simulink subsystem "currentControl"  (R2023b)
settings: Solver=VariableStepAuto  StartTime=0.0  StopTime=10.0  RelTol=1e-3
libraries: simulink x1
settings Model: Creator=jadam  LastModifiedBy=Veimar
settings DebuggingCC: UnconnectedInputMsg=warning  UnconnectedOutputMsg=warning  UnconnectedLineMsg=warning
settings ModelReferenceCC: EnableRefExpFcnMdlSchedulingChecks=on
settings RTWCC: DLArmComputeVersion=19.05

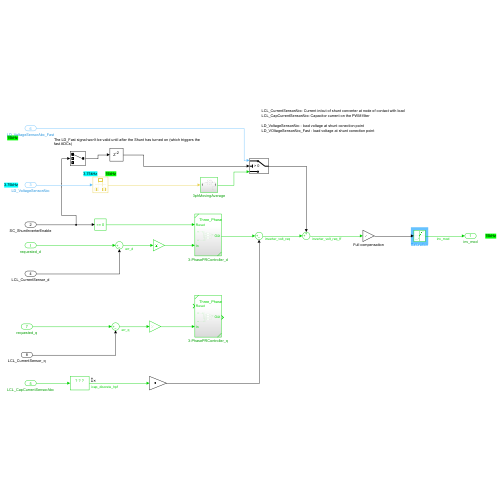
[thumbnail: Simulink's stored preview of the top-level diagram]
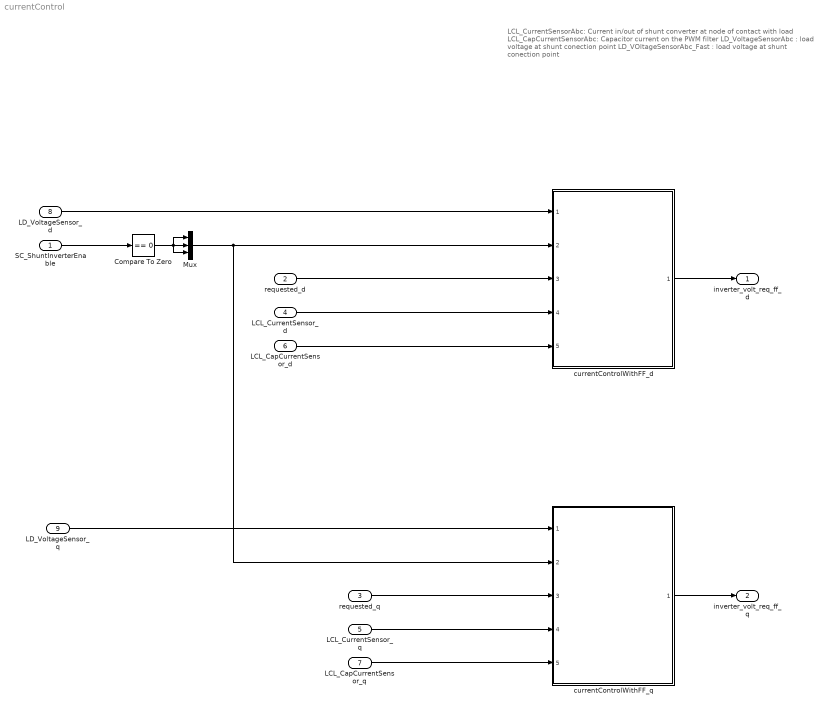
== system currentControl ==
  note: LCL_CurrentSensorAbc: Current in/out of shunt converter at node of contact with load
      | LCL_CapCurrentSensorAbc: Capacitor current on the PWM filter
      |
      | LD_VoltageSensorAbc : load voltage at shunt conection point
      | LD_VOltageSensorAbc_Fast : load voltage at shunt conection point
  SC_ShuntInverterEnable : Inport  OutDataTypeStr=boolean  PortDimensions=1
  requested_d : Inport  Port=2  OutDataTypeStr=single  PortDimensions=3
  requested_q : Inport  Port=3  OutDataTypeStr=single  PortDimensions=3
  LCL_CurrentSensor_d : Inport  Port=4  OutDataTypeStr=single  PortDimensions=3
  LCL_CurrentSensor_q : Inport  Port=5  OutDataTypeStr=single  PortDimensions=3
  LCL_CapCurrentSensor_d : Inport  Port=6  OutDataTypeStr=single  PortDimensions=3
  LCL_CapCurrentSensor_q : Inport  Port=7  OutDataTypeStr=single  PortDimensions=3
  LD_VoltageSensor_d : Inport  Port=8  OutDataTypeStr=single  PortDimensions=3
  LD_VoltageSensor_q : Inport  Port=9  OutDataTypeStr=single  PortDimensions=3
  Compare To Zero : simulink/Logic and Bit Operations/Compare To Zero  relop===  OutDataTypeStr=boolean
  Mux : Mux  Inputs=3
  currentControlWithFF_d : Subsystem  ReferencedSubsystem=currentControlWithFF
      settings: PermitHierarchicalResolution=None
  currentControlWithFF_q : Subsystem  ReferencedSubsystem=currentControlWithFF
      settings: PermitHierarchicalResolution=None
  inverter_volt_req_ff_d : Outport  OutDataTypeStr=single  PortDimensions=3
  inverter_volt_req_ff_q : Outport  Port=2  OutDataTypeStr=single  PortDimensions=3
  wires:
  SC_ShuntInverterEnable/1 -> Compare To Zero/1
  LD_VoltageSensor_d/1 -> currentControlWithFF_d/1
  Mux/1 -> currentControlWithFF_d/2, currentControlWithFF_q/2
  requested_d/1 -> currentControlWithFF_d/3
  LCL_CurrentSensor_d/1 -> currentControlWithFF_d/4
  LCL_CapCurrentSensor_d/1 -> currentControlWithFF_d/5
  requested_q/1 -> currentControlWithFF_q/3
  LCL_CurrentSensor_q/1 -> currentControlWithFF_q/4
  LCL_CapCurrentSensor_q/1 -> currentControlWithFF_q/5
  LD_VoltageSensor_q/1 -> currentControlWithFF_q/1
  currentControlWithFF_d/1 -> inverter_volt_req_ff_d/1
  currentControlWithFF_q/1 -> inverter_volt_req_ff_q/1
  Compare To Zero/1 -> Mux/2, Mux/1, Mux/3
